simulink model "check_ndtm_steer"  (R2018b)
settings: configuration reference "Physics" (kept outside this file)
libraries: simulink x2
settings Model: DataDictionary=check_ndtm.sldd  OrderedModelArguments=off  Creator=wischnewski  LastModifiedBy=ga25xiw

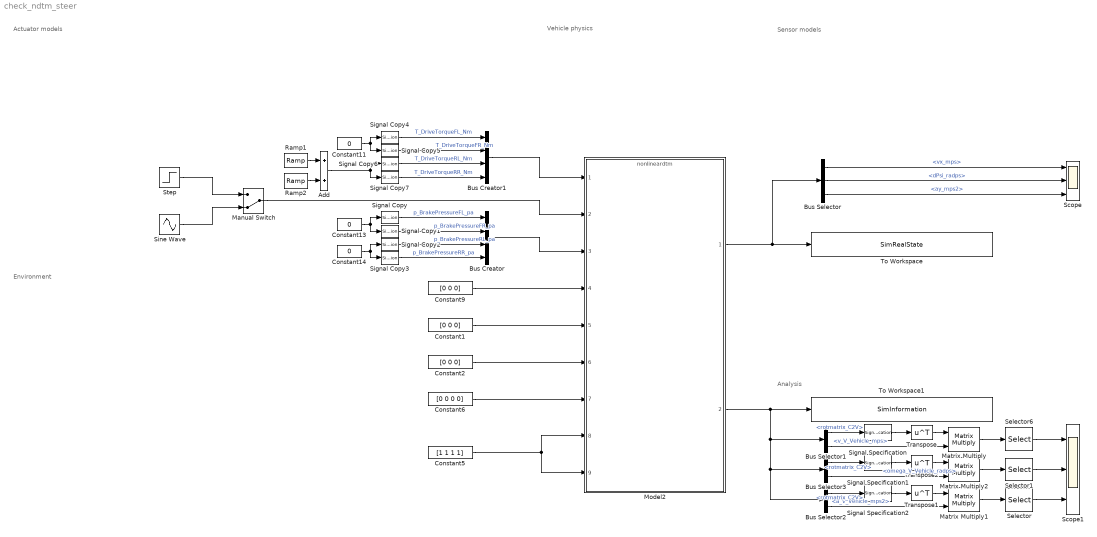
== system check_ndtm_steer ==
  note: Actuator models
  note: Vehicle physics
  note: Environment
  note: Analysis
  note: Sensor models
  Add : Sum
  Bus Creator : BusCreator  Inputs=4  OutDataTypeStr=Bus: BrakePressure_Pa
  Bus Creator1 : BusCreator  Inputs=4  OutDataTypeStr=Bus: DriveTorque_Nm
  Bus Selector : BusSelector  OutputSignals=vx_mps,dPsi_radps,ay_mps2
  Bus Selector1 : BusSelector  OutputSignals=Transformation.rotmatrix_C2V,Vehicle.v_V_Vehicle_mps
  Bus Selector2 : BusSelector  OutputSignals=Transformation.rotmatrix_C2V,Vehicle.a_V_Vehicle_mps2
  Bus Selector3 : BusSelector  OutputSignals=Transformation.rotmatrix_C2V,Vehicle.omega_V_Vehicle_radps
  Constant1 : Constant  Value=[0 0 0]
  Constant11 : Constant  Value=0
  Constant13 : Constant  Value=0
  Constant14 : Constant  Value=0
  Constant2 : Constant  Value=[0 0 0]
  Constant5 : Constant  Value=[1 1 1 1]
  Constant6 : Constant  Value=[0 0 0 0]
  Constant9 : Constant  Value=[0 0 0]
  Manual Switch : ManualSwitch  CurrentSetting=0
  Matrix Multiply : Product  Multiplication=Matrix(*)
  Matrix Multiply1 : Product  Multiplication=Matrix(*)
  Matrix Multiply2 : Product  Multiplication=Matrix(*)
  Model2 : ModelReference  ModelNameDialog=nonlineardtm  ParameterArgumentNames=x0_initialstates  ParameterArgumentValues=[0 0 0 0 0 -pi/2]  UsingDefaultArgumentValue=0  SimulationMode=Normal  ModelReferenceVersion=1.642
  Ramp1 : simulink/Sources/Ramp  slope=200  start=20  InitialOutput=0
  Ramp2 : simulink/Sources/Ramp  slope=-200  start=25  InitialOutput=0
  Scope : Scope  NumInputPorts=3
  Scope1 : Scope  NumInputPorts=3
  Selector : Selector  InputPortWidth=3  IndexOptions=Index vector (dialog)  Indices=2  OutputSizes=1
  Selector1 : Selector  InputPortWidth=3  IndexOptions=Index vector (dialog)  Indices=3  OutputSizes=1
  Selector6 : Selector  InputPortWidth=3  IndexOptions=Index vector (dialog)  Indices=1  OutputSizes=1
  Signal Copy{,1..7} (8 alike) : SignalConversion  OverrideOpt=off
  Signal Specification : SignalSpecification  Dimensions=[3 3]
  Signal Specification1 : SignalSpecification  Dimensions=[3 3]
  Signal Specification2 : SignalSpecification  Dimensions=[3 3]
  Sine Wave : Sin  Amplitude=0.5  Frequency=0.5  SampleTime=0
  Step : Step  Time=35  SampleTime=0
  To Workspace : ToWorkspace  VariableName=SimRealState  SaveFormat=Timeseries  SampleTime=-1
  To Workspace1 : ToWorkspace  VariableName=SimInformation  SaveFormat=Timeseries  SampleTime=-1
  Transpose : Math  Operator=transpose  SaturateOnIntegerOverflow=on
  Transpose1 : Math  Operator=transpose  SaturateOnIntegerOverflow=on
  Transpose2 : Math  Operator=transpose  SaturateOnIntegerOverflow=on
  wires:
  Bus Selector/1 -> Scope/1  "<vx_mps>"
  Bus Selector/2 -> Scope/2  "<dPsi_radps>"
  Bus Selector/3 -> Scope/3  "<ay_mps2>"
  Model2/1 -> Bus Selector/1, To Workspace/1
  Constant9/1 -> Model2/4
  Constant1/1 -> Model2/5
  Constant2/1 -> Model2/6
  Constant5/1 -> Model2/9, Model2/8
  Constant6/1 -> Model2/7
  Bus Selector1/1 -> Signal Specification/1  "<rotmatrix_C2V>"
  Transpose/1 -> Matrix Multiply/1
  Bus Selector1/2 -> Matrix Multiply/2  "<v_V_Vehicle_mps>"
  Matrix Multiply1/1 -> Selector/1
  Bus Selector2/2 -> Matrix Multiply1/2  "<a_V_Vehicle_mps2>"
  Transpose1/1 -> Matrix Multiply1/1
  Bus Selector2/1 -> Signal Specification2/1  "<rotmatrix_C2V>"
  Model2/2 -> Bus Selector2/1, Bus Selector3/1, Bus Selector1/1, To Workspace1/1
  Bus Selector3/1 -> Signal Specification1/1  "<rotmatrix_C2V>"
  Transpose2/1 -> Matrix Multiply2/1
  Bus Selector3/2 -> Matrix Multiply2/2  "<omega_V_Vehicle_radps>"
  Matrix Multiply/1 -> Selector6/1
  Selector/1 -> Scope1/3
  Selector1/1 -> Scope1/2
  Selector6/1 -> Scope1/1
  Signal Specification/1 -> Transpose/1
  Signal Specification1/1 -> Transpose2/1
  Signal Specification2/1 -> Transpose1/1
  Ramp1/1 -> Add/1
  Ramp2/1 -> Add/2
  Matrix Multiply2/1 -> Selector1/1
  Constant11/1 -> Signal Copy4/1, Signal Copy5/1
  Signal Copy6/1 -> Bus Creator1/3  "T_DriveTorqueRL_Nm"
  Signal Copy5/1 -> Bus Creator1/2  "T_DriveTorqueFR_Nm"
  Signal Copy7/1 -> Bus Creator1/4  "T_DriveTorqueRR_Nm"
  Signal Copy4/1 -> Bus Creator1/1  "T_DriveTorqueFL_Nm"
  Bus Creator1/1 -> Model2/1
  Constant14/1 -> Signal Copy3/1, Signal Copy2/1
  Constant13/1 -> Signal Copy1/1, Signal Copy/1
  Signal Copy2/1 -> Bus Creator/3  "p_BrakePressureRL_pa"
  Signal Copy1/1 -> Bus Creator/2  "p_BrakePressureFR_pa"
  Add/1 -> Signal Copy6/1, Signal Copy7/1
  Bus Creator/1 -> Model2/3
  Manual Switch/1 -> Model2/2
  Signal Copy3/1 -> Bus Creator/4  "p_BrakePressureRR_pa"
  Signal Copy/1 -> Bus Creator/1  "p_BrakePressureFL_pa"
  Sine Wave/1 -> Manual Switch/2
  Step/1 -> Manual Switch/1
